simulink model "HS"  (R2024b)
settings: Solver=VariableStepAuto  StartTime=0.0  StopTime=2  RelTol=1e-3
libraries: spsSeriesRLCBranchLib x6, spsDiodeLib x3, spsCurrentMeasurementLib x2, spsPVArrayLib x2, spsGroundLib x1, spsMosfetLib x1, spsPWMGeneratorDCDCLib x1, spsVoltageMeasurementLib x1, spspowerguiLib x1
settings Model: Creator=孙泽霖  LastModifiedBy=孙泽霖

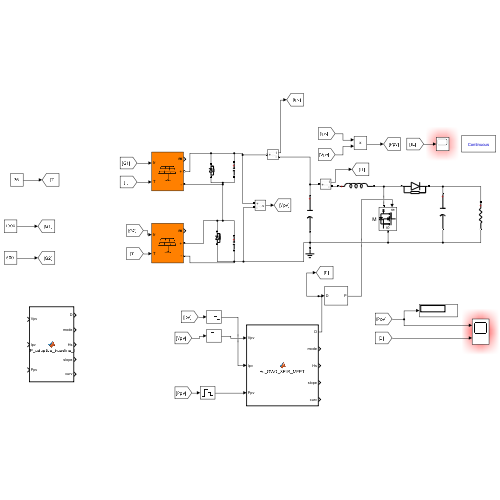
[thumbnail: Simulink's stored preview of the top-level diagram]
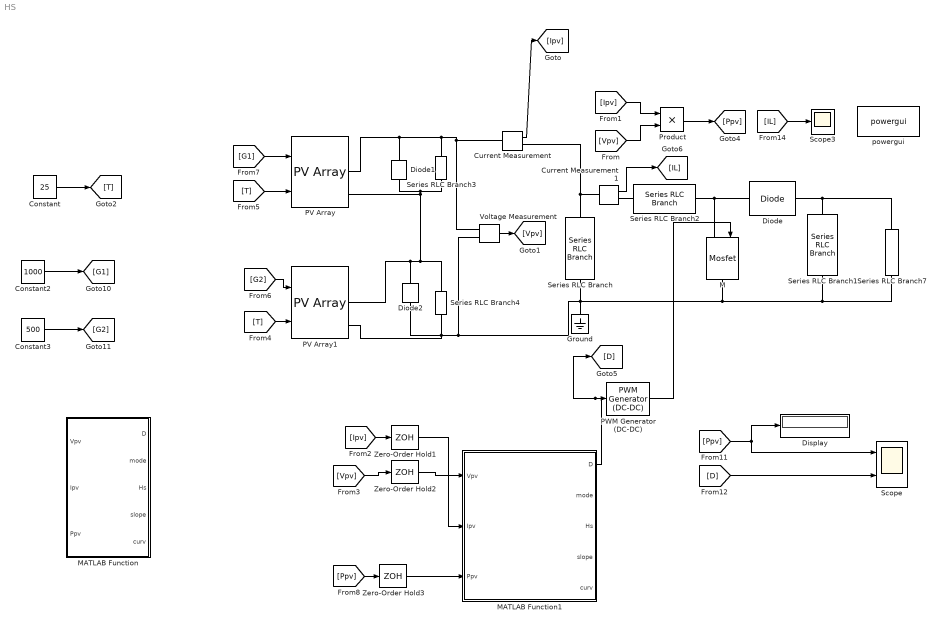
== system HS ==
  Constant : Constant  Value=25
  Constant2 : Constant  Value=1000
  Constant3 : Constant  Value=500
  Current Measurement : spsCurrentMeasurementLib/Current Measurement  PhasorSimulation=off  OutputType=Complex  PSBequivalent=0
  Current Measurement1 : spsCurrentMeasurementLib/Current Measurement  PhasorSimulation=off  OutputType=Complex  PSBequivalent=0
  Diode : spsDiodeLib/Diode  Ron=0.001  Lon=0  Vf=0.8  IC=0  UseSnubber=0  Rs=500  Cs=250e-9  Measurements=off
  Diode1 : spsDiodeLib/Diode  Ron=0.001  Lon=0  Vf=0.8  IC=0  UseSnubber=0  Rs=500  Cs=250e-9  Measurements=off
  Diode2 : spsDiodeLib/Diode  Ron=0.001  Lon=0  Vf=0.8  IC=0  UseSnubber=0  Rs=500  Cs=250e-9  Measurements=off
  Display : Display
  Ground : spsGroundLib/Ground  LConnTagsString=a
  M : spsMosfetLib/Mosfet  Ron=1e-3  Lon=0  Rd=1e-3  Vfd=0  IC=0  Rs=inf  Cs=inf  Measurements=off
  MATLAB Function : MATLAB Function  TreatAsAtomicUnit=on
  MATLAB Function1 : MATLAB Function  TreatAsAtomicUnit=on
  PV Array : spsPVArrayLib/PV Array  Npar=1  Nser=1  PlotType=array @ 1000 W/m2 & specified temperatures  S_vec="[ 1000  500  100 ]"  Temp_C_vec="[ 45 25  ]"  ModuleName=Kyocera Solar KC200GT  PlotWhenSelected=off  Pm=200.143  Ncell=54  Voc=32.9  Isc=8.21  Vm=26.3  Im=7.61  beta_Voc_pc=-0.355  alpha_Isc_pc=0.06  beta_Voc=-0.11679  alpha_Isc=0.004926  IL=8.2288  I0=2.3234e-10  nI=0.97734  Rsh=150.6844  Rs=0.34484  RobustModel=off  RobustCellTemperature=313.3991  BAL=on  Tc=1e-6  Tfilter=5e-5
  PV Array1 : spsPVArrayLib/PV Array  Npar=1  Nser=1  PlotType=array @ 1000 W/m2 & specified temperatures  S_vec="[ 1000  500  100 ]"  Temp_C_vec="[ 45 25  ]"  ModuleName=Kyocera Solar KC200GT  PlotWhenSelected=off  Pm=200.143  Ncell=54  Voc=32.9  Isc=8.21  Vm=26.3  Im=7.61  beta_Voc_pc=-0.355  alpha_Isc_pc=0.06  beta_Voc=-0.11679  alpha_Isc=0.004926  IL=8.2288  I0=2.3234e-10  nI=0.97734  Rsh=150.6844  Rs=0.34484  RobustModel=off  RobustCellTemperature=313.3991  BAL=on  Tc=1e-6  Tfilter=5e-5
  PWM Generator (DC-DC) : spsPWMGeneratorDCDCLib/PWM Generator (DC-DC)  Fsw=20000  Ts=0
  Product : Product
  Scope : Scope  NumInputPorts=2
  Scope3 : Scope
  Series RLC Branch : spsSeriesRLCBranchLib/Series RLC Branch  LConnTagsString=__new0  RConnTagsString=__new0  BranchType=C  Resistance=1  Inductance=1e-3  SetiL0=off  InitialCurrent=0  Capacitance=450e-6  Setx0=off  InitialVoltage=0  Measurements=None
  Series RLC Branch1 : spsSeriesRLCBranchLib/Series RLC Branch  LConnTagsString=__new0  RConnTagsString=__new0  BranchType=C  Resistance=0.1  Inductance=1e-3  SetiL0=off  InitialCurrent=0  Capacitance=500e-6  Setx0=off  InitialVoltage=0  Measurements=None
  Series RLC Branch2 : spsSeriesRLCBranchLib/Series RLC Branch  LConnTagsString=__new0  RConnTagsString=__new0  BranchType=L  Resistance=0.1  Inductance=65e-4  SetiL0=off  InitialCurrent=0  Capacitance=1e-6  Setx0=off  InitialVoltage=0  Measurements=None
  Series RLC Branch3 : spsSeriesRLCBranchLib/Series RLC Branch  LConnTagsString=__new0  RConnTagsString=__new0  BranchType=C  Resistance=1  Inductance=1e-3  SetiL0=off  InitialCurrent=0  Capacitance=100e-9  Setx0=off  InitialVoltage=0  Measurements=None
  Series RLC Branch4 : spsSeriesRLCBranchLib/Series RLC Branch  LConnTagsString=__new0  RConnTagsString=__new0  BranchType=C  Resistance=1  Inductance=1e-3  SetiL0=off  InitialCurrent=0  Capacitance=100e-9  Setx0=off  InitialVoltage=0  Measurements=None
  Series RLC Branch7 : spsSeriesRLCBranchLib/Series RLC Branch  LConnTagsString=__new0  RConnTagsString=__new0  BranchType=R  Resistance=44  Inductance=1e-3  SetiL0=off  InitialCurrent=0  Capacitance=400e-6  Setx0=off  InitialVoltage=0  Measurements=None
  Voltage Measurement : spsVoltageMeasurementLib/Voltage Measurement  PhasorSimulation=off  OutputType=Complex  PSBequivalent=0
  Zero-Order Hold1 : ZeroOrderHold  SampleTime=5e-4
  Zero-Order Hold2 : ZeroOrderHold  SampleTime=5e-4
  Zero-Order Hold3 : ZeroOrderHold  SampleTime=5e-4
  powergui : spspowerguiLib/powergui  Priority=1  SimulationMode=Continuous  SampleTime=1e-6  frequency=60  Iterations=50  frequencyindice=0  Pbase=100e6  ErrMax=1e-4  UnitsV=kV  UnitsW=MW  buscounter=0  FunctionMessages=off  echomessages=off  EnableUseOfTLC=off  CurrentSourceSwitches=off  DisableSnubberDevices=off  DisableRonSwitches=off  DisableVfSwitches=off  DisplayEquations=off  AutomaticDiscreteSolvers=off  SolverType=Tustin/Backward Euler (TBE)  Interpol=off  ExternalGateDelay=off  methode=off  Ts=100  x0status=blocks  SPID=on  SwTol=0  HookPort=off  NonlinearTolerance=1e-4  nMaxIteration=100  ContinueOnMaxIteration=off  RestoreLinks=warning  ResistiveCurrentMeasurement=off  Frange=[0:2:500]  Ylog=off  Xlog=on  ShowGrid=off  save=off  variable=ZData  structure=0  ZoomFFT=off  StartTime=0.0  cycles=1  DisplayStyle=1  fundamental=60  FreqAxis=off  MaxFrequency=1000  frequencyindicesteady=1  RmsSteady=1  display=off
  wires:
  Constant/1 -> [T]
  Current Measurement1/1 -> [IL]
  Constant3/1 -> [G2]
  [T] -> PV Array/2
  [G2] -> PV Array1/1
  Current Measurement/1 -> [Ipv]
  Voltage Measurement/1 -> [Vpv]
  [Vpv] -> Product/2
  [D] -> Scope/2
  [G1] -> PV Array/1
  Product/1 -> [Ppv]
  [IL] -> Scope3/1
  [Ppv] -> Display/1, Scope/1
  [Ipv] -> Product/1
  PWM Generator (DC-DC)/1 -> M/1
  Constant2/1 -> [G1]
  [T] -> PV Array1/2
  MATLAB Function1/1(D) -> [D], PWM Generator (DC-DC)/1
  [Ipv] -> Zero-Order Hold1/1
  [Vpv] -> Zero-Order Hold2/1
  Zero-Order Hold2/1 -> MATLAB Function1/1(Vpv)
  Zero-Order Hold1/1 -> MATLAB Function1/2(Ipv)
  [Ppv] -> Zero-Order Hold3/1
  Zero-Order Hold3/1 -> MATLAB Function1/3(Ppv)
  connections:
  Series RLC Branch2/RConn1 -- M/LConn1 -- Diode/LConn1
  Diode1/LConn1 -- Series RLC Branch3/RConn1 -- Series RLC Branch4/LConn1 -- Diode2/RConn1 -- PV Array1/RConn1 -- PV Array/RConn2
  Current Measurement/LConn1 -- Voltage Measurement/LConn1 -- Diode1/RConn1 -- PV Array/RConn1 -- Series RLC Branch3/LConn1
  Series RLC Branch/LConn1 -- Current Measurement1/LConn1 -- Current Measurement/RConn1
  Diode2/LConn1 -- PV Array1/RConn2 -- Series RLC Branch4/RConn1 -- Series RLC Branch/RConn1 -- M/RConn1 -- Series RLC Branch7/RConn1 -- Series RLC Branch1/RConn1 -- Ground/LConn1 -- Voltage Measurement/LConn2
  Series RLC Branch1/LConn1 -- Diode/RConn1 -- Series RLC Branch7/LConn1
  Current Measurement1/RConn1 -- Series RLC Branch2/LConn1

== matlab function HS/MATLAB Function1 ==
  data: Vpv input; D output; Ipv input; Ppv input; mode output; Hs output; slope output; curv output
function [D, mode, Hs, slope, curv] = Hs_GWO_SEIR_MPPT(Vpv, Ipv, Ppv)
%#codegen
% Hs-GWO-SEIR MPPT
% Shading-entropy guided Grey Wolf adaptive sampling and interval refinement MPPT
%
% 核心：
% 1. 用 GWO 生成自适应采样占空比；
% 2. 每个候选 D 测得 Pavg，并按 D 分箱构造 P-D 曲线；
% 3. 根据分箱 P-D 曲线计算遮荫熵 Hs；
% 4. Hs 反向控制 GWO 的收缩速度：
%       Hs低：曲线简单，快速向 Alpha 收缩；
%       Hs高：曲线复杂，保持 Alpha/Beta/Delta 多峰探索；
% 5. GWO 完成后，根据 Hs 保留 1/2/3 个候选区间；
% 6. 对候选区间进行局部细化扫描；
% 7. 最后进入小步局部 MPPT 微调。
%
% mode:
% -1 输入异常
%  1 局部稳态微调
%  2 普通局部跟踪
%  3 Hs较高，增强搜索
%  5 功率下降，反向
%  7 功率上升，快速跟踪
% 10 GWO自适应全局采样
% 20 候选区间细化
% 30 细化完成，跳到最终最佳点

%% ===================== 基本参数 =====================

Dmin = 0.12;
Dmax = 0.88;

% GWO 参数
PN = 6;              % 灰狼数量
MaxIter = 10;        % GWO最大迭代轮数

% 每个 GWO 候选点保持时间
HoldN_gwo   = 5;
SettleN_gwo = 1;

% D 分箱数量，用于构造 P-D 曲线和计算 Hs
BinN = 21;

% Hs 阈值
HsLow  = 0.25;
HsHigh = 0.55;

% 候选区间最大数量
MaxCand = 3;

% 候选区间细化参数
RefineN = 9;
HoldN_refine   = 7;
SettleN_refine = 2;

% 局部微调参数
HoldN_fast   = 8;
SettleN_fast = 2;

HoldN_slow   = 20;
SettleN_slow = 8;

stepMin   = 0.0004;
stepBase  = 0.0025;
stepAccel = 0.0012;

stepMaxLowHs  = 0.0100;
stepMaxHighHs = 0.0180;

% 功率判断死区
Pband = 0.20;

% 长期无提升后微启动
NoImproveLimit = 10;
ReboostStep = 0.0015;

% 功率低通系数
alphaP = 0.15;

%% ===================== 持久变量 =====================

persistent phase
persistent Dcur
persistent Pf

% 当前候选点保持采样
persistent sampleCounter
persistent Psum Pnum
persistent currentHoldN currentSettleN

% GWO 相关
persistent wolfD wolfP
persistent wolfIndex iterIndex

persistent Alpha_pos Alpha_score
persistent Beta_pos Beta_score
persistent Delta_pos Delta_score

persistent lastAlphaScore
persistent stableIter

% 分箱 P-D 曲线
persistent binPsum binCount Pbin

% 候选区间
persistent candCount candIndex
persistent candL candR

% 细化扫描
persistent refineIndex
persistent refineD refineP
persistent refineBestD refineBestP
persistent globalBestD globalBestP

% 输出观测量
persistent HsOut slopeOut curvOut slopePrev

% 局部微调
persistent hasPrev
persistent Pprev Dprev
persistent step lastDir
persistent successCount noImproveCount

persistent lastMode

if isempty(phase)

    phase = 10;

    Dcur = Dmin;
    Pf = Ppv;

    sampleCounter = 0;
    Psum = 0;
    Pnum = 0;
    currentHoldN = HoldN_gwo;
    currentSettleN = SettleN_gwo;

    wolfD = zeros(1, PN);
    wolfP = zeros(1, PN);

    % 初始灰狼均匀分布在全范围
    for i = 1:PN
        wolfD(i) = Dmin + (double(i) - 1) * (Dmax - Dmin) / double(PN - 1);
        wolfP(i) = 0;
    end

    wolfIndex = 1;
    iterIndex = 1;

    Dcur = wolfD(1);

    Alpha_pos = Dcur;
    Alpha_score = -1e9;

    Beta_pos = Dcur;
    Beta_score = -1e9;

    Delta_pos = Dcur;
    Delta_score = -1e9;

    lastAlphaScore = -1e9;
    stableIter = 0;

    binPsum = zeros(1, BinN);
    binCount = zeros(1, BinN);
    Pbin = zeros(1, BinN);

    candCount = 1;
    candIndex = 1;
    candL = zeros(1, MaxCand);
    candR = zeros(1, MaxCand);

    refineIndex = 1;
    refineD = zeros(1, RefineN);
    refineP = zeros(1, RefineN);

    refineBestD = Dcur;
    refineBestP = -1e9;

    globalBestD = Dcur;
    globalBestP = -1e9;

    HsOut = 0;
    slopeOut = 0;
    curvOut = 0;
    slopePrev = 0;

    hasPrev = false;
    Pprev = 0;
    Dprev = Dcur;

    step = stepBase;
    lastDir = 1;
    successCount = 0;
    noImproveCount = 0;

    lastMode = 10;
end

%% ===================== 输入保护 =====================

if ~isfinite(Vpv) || ~isfinite(Ipv) || ~isfinite(Ppv)
    D = Dcur;
    mode = -1;
    Hs = HsOut;
    slope = slopeOut;
    curv = curvOut;
    return;
end

if Ppv < 0
    Ppv = 0;
end

Pf = alphaP * Ppv + (1 - alphaP) * Pf;

%% ============================================================
% phase 10：GWO 自适应采样阶段
% ============================================================

if phase == 10

    sampleCounter = sampleCounter + 1;

    if sampleCounter > currentSettleN
        Psum = Psum + Pf;
        Pnum = Pnum + 1;
    end

    if sampleCounter < currentHoldN
        D = Dcur;
        mode = lastMode;
        Hs = HsOut;
        slope = slopeOut;
        curv = curvOut;
        return;
    end

    if Pnum > 0
        Pavg = Psum / double(Pnum);
    else
        Pavg = Pf;
    end

    sampleCounter = 0;
    Psum = 0;
    Pnum = 0;

    %% ---------- 记录当前灰狼适应度 ----------

    wolfP(wolfIndex) = Pavg;

    % 更新分箱 P-D 曲线
    ratio = (Dcur - Dmin) / (Dmax - Dmin);
    binIdx = floor(ratio * double(BinN - 1)) + 1;

    if binIdx < 1
        binIdx = 1;
    elseif binIdx > BinN
        binIdx = BinN;
    end

    binPsum(binIdx) = binPsum(binIdx) + Pavg;
    binCount(binIdx) = binCount(binIdx) + 1;

    % 更新 Alpha / Beta / Delta
    if Pavg > Alpha_score

        Delta_score = Beta_score;
        Delta_pos = Beta_pos;

        Beta_score = Alpha_score;
        Beta_pos = Alpha_pos;

        Alpha_score = Pavg;
        Alpha_pos = Dcur;

    elseif Pavg > Beta_score

        Delta_score = Beta_score;
        Delta_pos = Beta_pos;

        Beta_score = Pavg;
        Beta_pos = Dcur;

    elseif Pavg > Delta_score

        Delta_score = Pavg;
        Delta_pos = Dcur;
    end

    %% ---------- 继续测试当前迭代的下一只狼 ----------

    if wolfIndex < PN

        wolfIndex = wolfIndex + 1;
        Dcur = wolfD(wolfIndex);

        currentHoldN = HoldN_gwo;
        currentSettleN = SettleN_gwo;

        D = Dcur;
        mode = 10;
        Hs = HsOut;
        slope = slopeOut;
        curv = curvOut;
        lastMode = mode;
        return;
    end

    %% ---------- 一轮 GWO 结束，计算当前分箱 P-D 曲线和 Hs ----------

    for i = 1:BinN
        if binCount(i) > 0
            Pbin(i) = binPsum(i) / binCount(i);
        else
            Pbin(i) = 0;
        end
    end

    % 空箱简单补值
    for i = 1:BinN
        if Pbin(i) <= 0
            if i == 1
                Pbin(i) = Pbin(i+1);
            elseif i == BinN
                Pbin(i) = Pbin(i-1);
            else
                Pbin(i) = 0.5 * (Pbin(i-1) + Pbin(i+1));
            end
        end
    end

    totalDiff = 0;
    roughness = 0;
    signChange = 0;
    prevSign = 0;

    for i = 1:BinN-1
        dp = Pbin(i+1) - Pbin(i);
        totalDiff = totalDiff + abs(dp);

        if dp > Pband
            s = 1;
        elseif dp < -Pband
            s = -1;
        else
            s = 0;
        end

        if s ~= 0
            if prevSign ~= 0 && s ~= prevSign
                signChange = signChange + 1;
            end
            prevSign = s;
        end
    end

    for i = 1:BinN-2
        ddp = Pbin(i+2) - 2 * Pbin(i+1) + Pbin(i);
        roughness = roughness + abs(ddp);
    end

    if totalDiff > 1e-9
        roughRatio = roughness / totalDiff;
    else
        roughRatio = 0;
    end

    if roughRatio > 1
        roughRatio = 1;
    end

    signRatio = double(signChange) / double(BinN - 2);

    if signRatio > 1
        signRatio = 1;
    end

    HsOut = 0.6 * signRatio + 0.4 * roughRatio;

    if HsOut > 1
        HsOut = 1;
    elseif HsOut < 0
        HsOut = 0;
    end

    %% ---------- 判断是否提前稳定 ----------

    if abs(Alpha_score - lastAlphaScore) < 0.5
        stableIter = stableIter + 1;
    else
        stableIter = 0;
    end

    lastAlphaScore = Alpha_score;

    %% ---------- GWO 是否结束 ----------

    if iterIndex >= MaxIter || stableIter >= 3

        % 根据 Hs 决定保留几个候选峰区
        if HsOut < HsLow
            candCount = 1;
        elseif HsOut < HsHigh
            candCount = 2;
        else
            candCount = 3;
        end

        dBin = (Dmax - Dmin) / double(BinN - 1);

        % Hs越高，候选区间稍宽，避免漏峰
        if HsOut < HsLow
            halfW = 1.2 * dBin;
        elseif HsOut < HsHigh
            halfW = 1.8 * dBin;
        else
            halfW = 2.4 * dBin;
        end

        % 候选1：Alpha
        candL(1) = Alpha_pos - halfW;
        candR(1) = Alpha_pos + halfW;

        % 候选2：Beta
        candL(2) = Beta_pos - halfW;
        candR(2) = Beta_pos + halfW;

        % 候选3：Delta
        candL(3) = Delta_pos - halfW;
        candR(3) = Delta_pos + halfW;

        for i = 1:MaxCand
            if candL(i) < Dmin
                candL(i) = Dmin;
            end
            if candR(i) > Dmax
                candR(i) = Dmax;
            end
        end

        %% ---------- 初始化第一个候选区间细化 ----------

        candIndex = 1;

        for i = 1:RefineN
            refineD(i) = candL(1) + double(i - 1) * (candR(1) - candL(1)) / double(RefineN - 1);
            refineP(i) = 0;
        end

        refineIndex = 1;
        Dcur = refineD(1);

        refineBestP = -1e9;
        refineBestD = Dcur;

        globalBestP = -1e9;
        globalBestD = Dcur;

        phase = 20;

        currentHoldN = HoldN_refine;
        currentSettleN = SettleN_refine;

        D = Dcur;
        mode = 20;
        Hs = HsOut;
        slope = slopeOut;
        curv = curvOut;
        lastMode = mode;
        return;
    end

    %% ---------- Hs 控制 GWO 收缩速度 ----------

    aBase = 2.0 * (1.0 - double(iterIndex) / double(MaxIter));

    if aBase < 0
        aBase = 0;
    end

    % Hs越高，aEff越大，探索保持更久
    if HsOut < HsLow
        aEff = 0.55 * aBase;
        alphaBlend = 0.45;   % 低熵：更快向 Alpha 收缩
    elseif HsOut < HsHigh
        aEff = 0.75 * aBase;
        alphaBlend = 0.25;
    else
        aEff = 1.00 * aBase;
        alphaBlend = 0.10;   % 高熵：慢收缩，保留多峰探索
    end

    %% ---------- 更新狼群位置 ----------

    for i = 1:PN

        % 伪随机数，避免 codegen 下随机种子问题
        r1 = abs(sin(double(iterIndex * 13 + i * 7 + 1)));
        r2 = abs(sin(double(iterIndex * 17 + i * 5 + 2)));

        A1 = 2.0 * aEff * r1 - aEff;
        C1 = 2.0 * r2;

        D_alpha = abs(C1 * Alpha_pos - wolfD(i));
        X1 = Alpha_pos - A1 * D_alpha;

        r1 = abs(sin(double(iterIndex * 19 + i * 11 + 3)));
        r2 = abs(sin(double(iterIndex * 23 + i * 3 + 4)));

        A2 = 2.0 * aEff * r1 - aEff;
        C2 = 2.0 * r2;

        D_beta = abs(C2 * Beta_pos - wolfD(i));
        X2 = Beta_pos - A2 * D_beta;

        r1 = abs(sin(double(iterIndex * 29 + i * 13 + 5)));
        r2 = abs(sin(double(iterIndex * 31 + i * 17 + 6)));

        A3 = 2.0 * aEff * r1 - aEff;
        C3 = 2.0 * r2;

        D_delta = abs(C3 * Delta_pos - wolfD(i));
        X3 = Delta_pos - A3 * D_delta;

        newD = (X1 + X2 + X3) / 3.0;

        % Hs低时向Alpha更快靠拢；Hs高时少量靠拢，保留探索
        newD = (1.0 - alphaBlend) * newD + alphaBlend * Alpha_pos;

        if newD < Dmin
            newD = Dmin;
        elseif newD > Dmax
            newD = Dmax;
        end

        wolfD(i) = newD;
        wolfP(i) = 0;
    end

    iterIndex = iterIndex + 1;
    wolfIndex = 1;
    Dcur = wolfD(1);

    currentHoldN = HoldN_gwo;
    currentSettleN = SettleN_gwo;

    D = Dcur;
    mode = 10;
    Hs = HsOut;
    slope = slopeOut;
    curv = curvOut;
    lastMode = mode;
    return;
end

%% ============================================================
% phase 20：候选区间细化扫描
% ============================================================

if phase == 20

    sampleCounter = sampleCounter + 1;

    if sampleCounter > currentSettleN
        Psum = Psum + Pf;
        Pnum = Pnum + 1;
    end

    if sampleCounter < currentHoldN
        D = Dcur;
        mode = lastMode;
        Hs = HsOut;
        slope = slopeOut;
        curv = curvOut;
        return;
    end

    if Pnum > 0
        Pavg2 = Psum / double(Pnum);
    else
        Pavg2 = Pf;
    end

    sampleCounter = 0;
    Psum = 0;
    Pnum = 0;

    refineP(refineIndex) = Pavg2;

    if Pavg2 > refineBestP
        refineBestP = Pavg2;
        refineBestD = Dcur;
    end

    if refineIndex < RefineN

        refineIndex = refineIndex + 1;
        Dcur = refineD(refineIndex);

        currentHoldN = HoldN_refine;
        currentSettleN = SettleN_refine;

        D = Dcur;
        mode = 20;
        Hs = HsOut;
        slope = slopeOut;
        curv = curvOut;
        lastMode = mode;
        return;
    end

    %% ---------- 当前候选区间细化完成 ----------

    if refineBestP > globalBestP
        globalBestP = refineBestP;
        globalBestD = refineBestD;
    end

    if candIndex < candCount

        candIndex = candIndex + 1;

        for i = 1:RefineN
            refineD(i) = candL(candIndex) + double(i - 1) * (candR(candIndex) - candL(candIndex)) / double(RefineN - 1);
            refineP(i) = 0;
        end

        refineIndex = 1;
        Dcur = refineD(1);

        refineBestP = -1e9;
        refineBestD = Dcur;

        currentHoldN = HoldN_refine;
        currentSettleN = SettleN_refine;

        D = Dcur;
        mode = 20;
        Hs = HsOut;
        slope = slopeOut;
        curv = curvOut;
        lastMode = mode;
        return;

    else

        %% ---------- 所有候选区间细化完成，进入局部微调 ----------

        Dcur = globalBestD;
        phase = 2;

        hasPrev = false;
        Pprev = 0;
        Dprev = Dcur;

        step = stepBase;
        successCount = 0;
        noImproveCount = 0;

        if Dcur > (Dmin + Dmax) / 2
            lastDir = -1;
        else
            lastDir = 1;
        end

        currentHoldN = HoldN_fast;
        currentSettleN = SettleN_fast;

        D = Dcur;
        mode = 30;
        Hs = HsOut;
        slope = slopeOut;
        curv = curvOut;
        lastMode = mode;
        return;
    end
end

%% ============================================================
% phase 2：局部微调
% ============================================================

sampleCounter = sampleCounter + 1;

if sampleCounter > currentSettleN
    Psum = Psum + Pf;
    Pnum = Pnum + 1;
end

if sampleCounter < currentHoldN
    D = Dcur;
    mode = lastMode;
    Hs = HsOut;
    slope = slopeOut;
    curv = curvOut;
    return;
end

if Pnum > 0
    Plocal = Psum / double(Pnum);
else
    Plocal = Pf;
end

sampleCounter = 0;
Psum = 0;
Pnum = 0;

if ~hasPrev

    Pprev = Plocal;
    Dprev = Dcur;
    hasPrev = true;

    Dcandidate = Dcur + lastDir * step;

    if Dcandidate > Dmax
        Dcandidate = Dmax;
        lastDir = -1;
    elseif Dcandidate < Dmin
        Dcandidate = Dmin;
        lastDir = 1;
    end

    Dcur = Dcandidate;

    D = Dcur;
    mode = 2;
    Hs = HsOut;
    slope = slopeOut;
    curv = curvOut;
    lastMode = mode;
    return;
end

dP = Plocal - Pprev;
dD = Dcur - Dprev;

if abs(dD) > 1e-9
    slopeNow = dP / dD;
else
    slopeNow = slopePrev;
end

if abs(dD) > 1e-9
    curvNow = (slopeNow - slopePrev) / dD;
else
    curvNow = 0;
end

slopeOut = slopeNow;
curvOut = curvNow;

if HsOut > HsHigh
    stepMax = stepMaxHighHs;
else
    stepMax = stepMaxLowHs;
end

modeNow = 2;
dir = lastDir;

if dP > Pband

    dir = lastDir;
    successCount = successCount + 1;
    noImproveCount = 0;

    step = stepBase + stepAccel * double(successCount);

    if step > stepMax
        step = stepMax;
    end

    if HsOut > HsHigh
        modeNow = 3;
    else
        modeNow = 7;
    end

elseif dP < -Pband

    dir = -lastDir;
    successCount = 0;

    step = step * 0.5;

    if step < stepMin
        step = stepMin;
    end

    modeNow = 5;

else

    successCount = 0;
    noImproveCount = noImproveCount + 1;

    dir = lastDir;
    step = stepMin;
    modeNow = 1;

    if noImproveCount >= NoImproveLimit
        step = ReboostStep;
        noImproveCount = 0;

        if HsOut > HsHigh
            modeNow = 3;
        else
            modeNow = 2;
        end
    end
end

% Hs 对局部阶段的附加调节
if HsOut > HsHigh

    if step > stepMaxHighHs
        step = stepMaxHighHs;
    end

elseif HsOut > HsLow

    if dP > Pband
        step = step * 1.10;
        if step > stepMax
            step = stepMax;
        end
    end

else

    if step > stepMaxLowHs
        step = stepMaxLowHs;
    end
end

Dcandidate = Dcur + dir * step;

if Dcandidate > Dmax
    Dcandidate = Dmax;
    lastDir = -1;
elseif Dcandidate < Dmin
    Dcandidate = Dmin;
    lastDir = 1;
else
    if dir > 0
        lastDir = 1;
    elseif dir < 0
        lastDir = -1;
    end
end

if modeNow == 7
    currentHoldN = HoldN_fast;
    currentSettleN = SettleN_fast;
elseif modeNow == 3 || modeNow == 5 || modeNow == 1
    currentHoldN = HoldN_slow;
    currentSettleN = SettleN_slow;
else
    if step >= 0.004
        currentHoldN = HoldN_fast;
        currentSettleN = SettleN_fast;
    else
        currentHoldN = HoldN_slow;
        currentSettleN = SettleN_slow;
    end
end

Dprev = Dcur;
Pprev = Plocal;
slopePrev = slopeNow;

Dcur = Dcandidate;

D = Dcur;
mode = modeNow;
Hs = HsOut;
slope = slopeOut;
curv = curvOut;

lastMode = modeNow;

end

== matlab function HS/MATLAB Function ==
  data: Vpv input; D output; Ipv input; Ppv input; mode output; Hs output; slope output; curv output
function [D, mode, Hs, slope, curv] = SECP_adaptive_baseline_lock(Vpv, Ipv, Ppv)
%#codegen
% SECP-adaptive baseline MPPT with peak-lock
% Continuous powergui + discrete ZOH sampling

%% ===================== 基本参数 =====================

D0   = 0.50;
Dmin = 0.20;
Dmax = 0.80;

dD_min   = 0.0001;
dD_base  = 0.00025;
dD_max   = 0.0012;

P_dead = 0.10;
V_dead = 0.02;

alpha = 0.05;

Nwin = 10;

Hs_low  = 0.25;
Hs_high = 0.55;

curv_th = 0.5;

HoldLimit = 8;

% 峰值锁定参数
P_drop   = 0.5;    % 若功率等级较小，可改成0.2；若功率很大，可改成1
LockGain = 0.5;    % 0.3更柔和，0.8更快拉回
DropLimit = 3;     % 连续几次下降后触发锁定

%% ===================== 持久变量 =====================

persistent Dold Vold Pold
persistent Vf If Pf
persistent slope_old
persistent Pbuf Vbuf idx count
persistent lastDir
persistent holdCounter
persistent Pbest Dbest dropCounter

if isempty(Dold)
    Dold = D0;

    Vf = Vpv;
    If = Ipv;
    Pf = Ppv;

    Vold = Vpv;
    Pold = Ppv;

    slope_old = 0;

    Pbuf = zeros(1, Nwin);
    Vbuf = zeros(1, Nwin);
    idx = 1;
    count = 0;

    lastDir = 1;
    holdCounter = 0;

    Pbest = 0;
    Dbest = D0;
    dropCounter = 0;
end

%% ===================== 输入保护 =====================

if ~isfinite(Vpv) || ~isfinite(Ipv) || ~isfinite(Ppv)
    D = Dold;
    mode = -1;
    Hs = 0;
    slope = 0;
    curv = 0;
    return;
end

if Vpv < 0
    Vpv = 0;
end

if Ipv < 0
    Ipv = 0;
end

if Ppv < 0
    Ppv = 0;
end

%% ===================== 低通滤波 =====================

Vf = alpha * Vpv + (1 - alpha) * Vf;
If = alpha * Ipv + (1 - alpha) * If;
Pf = alpha * Ppv + (1 - alpha) * Pf;

%% ===================== 更新历史最佳点 =====================

if Pf > Pbest
    Pbest = Pf;
    Dbest = Dold;
    dropCounter = 0;
end

%% ===================== 更新窗口 =====================

Pbuf(idx) = Pf;
Vbuf(idx) = Vf;

idx = idx + 1;
if idx > Nwin
    idx = 1;
end

if count < Nwin
    count = count + 1;
end

%% ===================== 计算 dP/dV 和曲率 =====================

dV = Vf - Vold;
dP = Pf - Pold;

if abs(dV) < 1e-6
    slope = slope_old;
else
    slope = dP / dV;
end

if abs(dV) < 1e-6
    curv = 0;
else
    curv = (slope - slope_old) / dV;
end

%% ===================== 计算 Hs =====================

Hs = 0;

if count >= Nwin
    Ptemp = zeros(1, Nwin);

    for i = 1:Nwin
        pos = idx + i - 1;
        if pos > Nwin
            pos = pos - Nwin;
        end
        Ptemp(i) = Pbuf(pos);
    end

    dPsum = 0;
    dParr = zeros(1, Nwin - 1);

    for i = 1:Nwin - 1
        dParr(i) = abs(Ptemp(i + 1) - Ptemp(i));
        dPsum = dPsum + dParr(i);
    end

    if dPsum > 1e-9
        Htemp = 0;

        for i = 1:Nwin - 1
            q = dParr(i) / dPsum;
            if q > 1e-12
                Htemp = Htemp - q * log(q);
            end
        end

        Hs = Htemp / log(double(Nwin - 1));
    else
        Hs = 0;
    end
else
    Hs = 0;
end

%% ===================== 数据不足阶段 =====================

if count < Nwin
    D = Dold;
    mode = 0;

    Vold = Vf;
    Pold = Pf;
    slope_old = slope;
    return;
end

%% ===================== 自适应步长 =====================

slope_norm = abs(slope) / (abs(slope) + 1);
curv_norm  = abs(curv)  / (abs(curv)  + 1);

dD = dD_base;

dD = dD + 0.00025 * slope_norm;

if Hs > Hs_high
    dD = dD + 0.00035;
elseif Hs > Hs_low
    dD = dD + 0.00015;
end

if abs(curv) > curv_th && abs(slope) < 5
    dD = dD * 0.5;
end

if dD > dD_max
    dD = dD_max;
elseif dD < dD_min
    dD = dD_min;
end

%% ===================== 主方向判断 =====================

if abs(dP) < P_dead && abs(dV) < V_dead
    dir = 0;
    mode = 1;
else
    if dP > 0
        dir = lastDir;
    elseif dP < 0
        dir = -lastDir;
    else
        dir = lastDir;
    end

    if Hs > Hs_high
        mode = 3;
    else
        mode = 2;
    end
end

%% ===================== 防卡死但不漂移 =====================

if dir == 0
    holdCounter = holdCounter + 1;
else
    holdCounter = 0;
end

if holdCounter >= HoldLimit
    % 不再强制沿lastDir扰动，防止越过MPP后继续漂移
    dir = 0;
    dD = dD_min;
    holdCounter = 0;
    mode = 1;
end

%% ===================== 曲率辅助减小步长 =====================

if abs(slope) < 2 && curv < -curv_th
    dD = dD_min;
end

%% ===================== 峰值锁定机制 =====================

if Pf < Pbest - P_drop
    dropCounter = dropCounter + 1;
else
    dropCounter = 0;
end

if dropCounter >= DropLimit
    % 当前功率已经明显低于历史最优，向Dbest回拉
    Dnew = Dold + LockGain * (Dbest - Dold);
    mode = 4;

    % 防止下一步继续沿错误方向漂移
    if Dbest > Dold
        lastDir = 1;
    elseif Dbest < Dold
        lastDir = -1;
    end

    dropCounter = 0;
else
    Dnew = Dold + dir * dD;
end

%% ===================== 占空比限幅 =====================

if Dnew > Dmax
    Dnew = Dmax;
    lastDir = -1;
elseif Dnew < Dmin
    Dnew = Dmin;
    lastDir = 1;
else
    if dir > 0
        lastDir = 1;
    elseif dir < 0
        lastDir = -1;
    end
end

%% ===================== 状态更新 =====================

Dold = Dnew;
Vold = Vf;
Pold = Pf;
slope_old = slope;

D = Dold;

end
